simulink model "pid2_1"  (R2017b)
settings: Solver=FixedStepAuto  StartTime=0.0  StopTime=10.0  FixedStep=0.1  RelTol=1e-3
libraries: neural x93
(part 3 of 3)

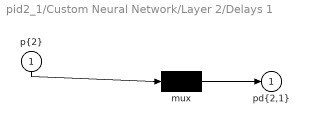
== system pid2_1/Custom Neural Network/Layer 2/Delays 1 ==
  "p{2}" : Inport  PortDimensions=90  SampleTime=0.1
      mask Display: e = 0.06;c1 = [120 230 180]/255;c2 = ([120 230 180]+0)/(256+128);c3 = ([120 230 180]+128)/(256+128);patch([0 1 1 0],[0 0 1 1],c1);patch([0 1 1 1-e 1-e 0+e],[0 0 1 1-e 0+e 0+e],c2);patch([0 0 1 1-e 0+e 0+e],[0 1 1 1-e 1-e 0+e],c3);plot([0 1 1 0 0],[0 0 1 1 0]);
  mux : Mux  Inputs=1
      mask Display: e = 0.06;c1 = [120 150 230]/255;c2 = ([120 150 230]+0)/383;c3 = ([120 150 230]+128)/383;patch([0 1 1 0],[0 0 1 1],c1);patch([0 1 1 1-e 1-e 0+e],[0 0 1 1-e 0+e 0+e],c2);patch([0 0 1 1-e 0+e 0+e],[0 1 1 1-e 1-e 0+e],c3);plot([0 1 1 0 0],[0 0 1 1 0]);disp('Mux')
  "pd{2,1}" : Outport
      mask Display: e = 0.06;c1 = [120 230 180]/255;c2 = ([120 230 180]+0)/(256+128);c3 = ([120 230 180]+128)/(256+128);patch([0 1 1 0],[0 0 1 1],c1);patch([0 1 1 1-e 1-e 0+e],[0 0 1 1-e 0+e 0+e],c2);patch([0 0 1 1-e 0+e 0+e],[0 1 1 1-e 1-e 0+e],c3);plot([0 1 1 0 0],[0 0 1 1 0]);
  wires:
  "p{2}"/1 -> mux/1
  mux/1 -> "pd{2,1}"/1

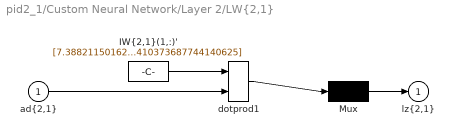
== system pid2_1/Custom Neural Network/Layer 2/LW{2,1} ==
  "ad{2,1}" : Inport  PortDimensions=90  SampleTime=0.1
      mask Display: e = 0.06;c1 = [120 230 180]/255;c2 = ([120 230 180]+0)/(256+128);c3 = ([120 230 180]+128)/(256+128);patch([0 1 1 0],[0 0 1 1],c1);patch([0 1 1 1-e 1-e 0+e],[0 0 1 1-e 0+e 0+e],c2);patch([0 0 1 1-e 0+e 0+e],[0 1 1 1-e 1-e 0+e],c3);plot([0 1 1 0 0],[0 0 1 1 0]);
  "IW{2,1}(1,:)'" : Constant  Value=[7.38821150162222206603246377198956906795501708984375;-3.31834809174878397897145987371914088726043701171875;-16.918699271172425113718418288044631481170654296875;9.707415219320392196777902427129447460174560546875;-11.204331487007575418601845740340650081634521484375;-0.93171519503237554271635190161759965121746063232421875;6.97340106077758292713042465038597583770751953125;6.79688995083058511426088443840853869915008544921875;-6.64210914260966323041657233261503279209136962890625;38.16514526502250959083539783023297786712646484375;-1.2997168442302886592898403250728733837604522705078125;-10.8674232133649031339928114903159439563751220703125;-7.53145315235564805078638528357259929180145263671875;-35.8624718982225232366545242257416248321533203125;1.62707826256527798847173471585847437381744384765625;7.34711134477760907657284406013786792755126953125;-38.76933099101463398028499796055257320404052734375;7.0101997481068991646679933182895183563232421875;-1.0800272242546540280017097757081501185894012451171875;7.22268603902242478653761281748302280902862548828125;-31.908603932248372103686051559634506702423095703125;31.43801439379043216604259214363992214202880859375;-0.6850933378908530269058019257499836385250091552734375;7.1846569151794756891149518196471035480499267578125;37.666813071511313637529383413493633270263671875;-37.44516457141643428485622280277311801910400390625;7.24509178494552319449439892196096479892730712890625;-37.85842583666080685134147643111646175384521484375;-12.0265672962244831722955495934002101421356201171875;7.67646638627952970779233510256744921207427978515625;-6.42448220135708414346709105302579700946807861328125;10.3331049660226081954306209809146821498870849609375;-3.008244122054132052568320432328619062900543212890625;1.2082065343981327476541309806634671986103057861328125;37.68470332901879515929977060295641422271728515625;0.7058554061668360635195540453423745930194854736328125;-0.67079172199094638795457967717084102332592010498046875;24.687279509380065434243078925646841526031494140625;5.3779333205647628091128353844396770000457763671875;-1.1388340317662801748355150266434065997600555419921875;-7.34333694386511570684206162695772945880889892578125;7.6687901277150398726689672912470996379852294921875;37.039238895939803342116647399961948394775390625;-0.74886079065950672539742072331137023866176605224609375;-6.50129995516258674115306348539888858795166015625;-1.1508423954399751298893761486397124826908111572265625;-5.34378874119396574116080955718643963336944580078125;-7.18734326094112674354619230143725872039794921875;-0.351285576349237349536025476481881923973560333251953125;-1.557067976755823313084192704991437494754791259765625;-7.5389206613684240920747470227070152759552001953125;-7.121917853448277213601613766513764858245849609375;7.28547335190423428485928525333292782306671142578125;-3.175186510198348965872128246701322495937347412109375;7.2690982220764919219391231308691203594207763671875;-3.4326283662708920729755845968611538410186767578125;-3.309111676044532490692517967545427381992340087890625;-7.04667592491648964170281033148057758808135986328125;7.5223993048423540841440626536495983600616455078125;0.769061050988695260599570246995426714420318603515625;37.8811160550852719097747467458248138427734375;-18.084920414470335714440807350911200046539306640625;7.35841504648805777577535991440527141094207763671875;-1.2445708307753633459213915557484142482280731201171875;15.4731082227877312362807060708291828632354736328125;-9.7010049482701621315072770812548696994781494140625;-5.5023205769554124344722367823123931884765625;37.73344018197980176410055719316005706787109375;6.95149116010535284004845379968173801898956298828125;5.8496005690000512089454787201248109340667724609375;37.72765436371188485509264864958822727203369140625;-8.426148553956625875116515089757740497589111328125;-14.2177713222957446959071603487245738506317138671875;0.56220107818503184393676974650588817894458770751953125;-29.275827405182294427277156501077115535736083984375 ...(+800 chars)]
      mask Display: e = 0.06;c1 = [120 150 230]/255;c2 = ([120 150 230]+0)/383;c3 = ([120 150 230]+128)/383;patch([0 1 1 0],[0 0 1 1],c1);patch([0 1 1 1-e 1-e 0+e],[0 0 1 1-e 0+e 0+e],c2);patch([0 0 1 1-e 0+e 0+e],[0 1 1 1-e 1-e 0+e],c3);plot([0 1 1 0 0],[0 0 1 1 0]);disp('weights');
  Mux : Mux  Inputs=1
      mask Display: e = 0.06;c1 = [120 150 230]/255;c2 = ([120 150 230]+0)/383;c3 = ([120 150 230]+128)/383;patch([0 1 1 0],[0 0 1 1],c1);patch([0 1 1 1-e 1-e 0+e],[0 0 1 1-e 0+e 0+e],c2);patch([0 0 1 1-e 0+e 0+e],[0 1 1 1-e 1-e 0+e],c3);plot([0 1 1 0 0],[0 0 1 1 0]);disp('Mux');
  dotprod1 : neural/Weight Functions/dotprod
  "lz{2,1}" : Outport
      mask Display: e = 0.06;c1 = [120 230 180]/255;c2 = ([120 230 180]+0)/(256+128);c3 = ([120 230 180]+128)/(256+128);patch([0 1 1 0],[0 0 1 1],c1);patch([0 1 1 1-e 1-e 0+e],[0 0 1 1-e 0+e 0+e],c2);patch([0 0 1 1-e 0+e 0+e],[0 1 1 1-e 1-e 0+e],c3);plot([0 1 1 0 0],[0 0 1 1 0]);
  wires:
  "IW{2,1}(1,:)'"/1 -> dotprod1/1
  "ad{2,1}"/1 -> dotprod1/2
  dotprod1/1 -> Mux/1
  Mux/1 -> "lz{2,1}"/1
